simulink model "task3"  (R2023b)
settings: Solver=FixedStepDiscrete  StartTime=0.0  StopTime=10.0  FixedStep=5e-5  RelTol=1e-3
PreLoadFcn:
  | Simulink.defineIntEnumType('windowCommand', {'Off','Speed1','Speed2','Speed3'},[0,1,2,3])
libraries: simulink x1, fuzblock x1, slctrl_autotuning x1, slpidlib x1
settings Model: Creator=kz1nz0  LastModifiedBy=Ja

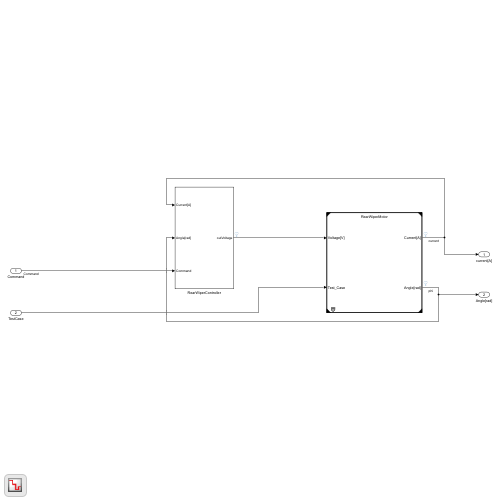
[thumbnail: Simulink's stored preview of the top-level diagram]
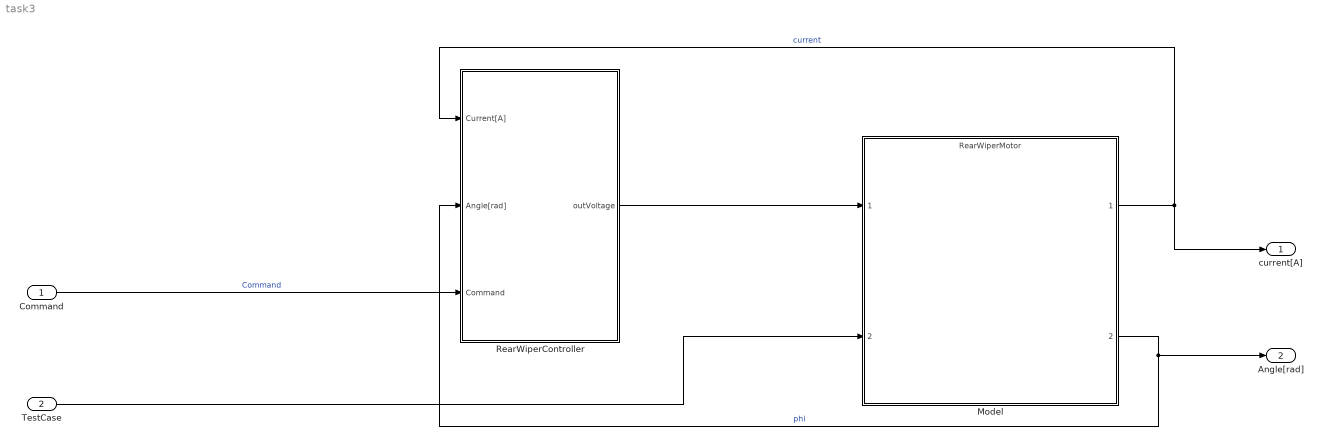
== system task3 ==
  Command : Inport  OutDataTypeStr=Enum: windowCommand
  TestCase : Inport  Port=2  OutDataTypeStr=int8
  Model : ModelReference  ModelNameDialog=RearWiperMotor.slxp  ModelReferenceVersion=19.15  CopyOfModelProtected=on
  RearWiperController : Subsystem
  current[A] : Outport
  Angle[rad] : Outport  Port=2
  wires:
  Command/1 -> RearWiperController/3(Command)  "Command"
  TestCase/1 -> Model/2
  Model/1 -> current[A]/1, RearWiperController/1(Current[A])  "current"
  Model/2 -> RearWiperController/2(Angle[rad]), Angle[rad]/1  "phi"
  RearWiperController/1(outVoltage) -> Model/1

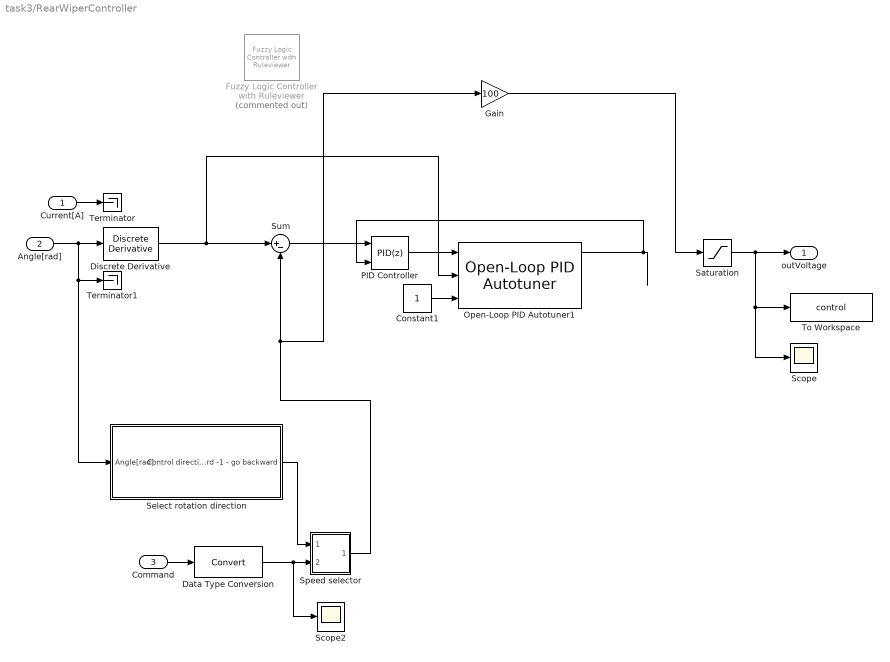
== system task3/RearWiperController ==
  Current[A] : Inport
  Angle[rad] : Inport  Port=2
  Command : Inport  Port=3  OutDataTypeStr=Enum: windowCommand
  Constant1 : Constant
  Data Type Conversion : DataTypeConversion  SaturateOnIntegerOverflow=off  RndMeth=Floor
  Discrete Derivative : simulink/Quick Insert/Discrete/Discrete Derivative  gainval=1.0  ICPrevScaledInput=0.0  OutMin=[]  OutMax=[]  OutDataType=fixdt(1, 16)  OutScaling=2^-10  DoSatur=off
  Fuzzy Logic Controller with Ruleviewer : fuzblock/Fuzzy Logic  Controller  with Ruleviewer  Commented=on  fismatrix=fis  Ts=2
  Gain : Gain  Gain=100
  Open-Loop PID Autotuner1 : slctrl_autotuning/Open-Loop PID Autotuner  PIDType=PID  PIDForm=Parallel  TimeDomain=discrete-time  DiscreteTs=5e-5  IntegratorFormula=Forward Euler  FilterFormula=Forward Euler  ContinuousTs=0.02  Bandwidth=1  UseExternalWC=off  TargetPM=60  UseExternalPM=off  UseExternalAchievedPM=off  AmpSine=1  UseExternalAmpSine=off  EstimateDCGain=on  AmpStep=1  UseExternalAmpStep=off  UseExternalFRD=off  UseExternalU0=off  UseExternalDCGain=off  NotDeployTuningModule=off  UsePLCCoder=off  BlockDataType=double  UseConnectedPID=on  blockpath=[]  tunedP=0  tunedI=0  tunedD=0  tunedN=100  tunedPM=0  EstimationWindowSize=3
      settings: LibrarySourceBlock=slctrlblks/Autotuning/Open-Loop PID Autotuner
  PID Controller : slpidlib/PID Controller  Controller=PID  Form=Parallel  TimeDomain=Discrete-time  UseExternalTs=off  SampleTime=-1  IntegratorMethod=Forward Euler  FilterMethod=Forward Euler  ControllerParametersSource=internal  P=100  I=1  UseKiTs=off  D=1  N=100  UseFilter=on  TunerSelectOption=Transfer Function Based (PID Tuner App)  InitialConditionSource=internal  InitialConditionForIntegrator=0  InitialConditionForFilter=0  DifferentiatorICPrevScaledInput=0  ExternalReset=none  TrackingMode=on  Kt=1  LimitOutput=off  SatLimitsSource=internal  UpperSaturationLimit=inf  LowerSaturationLimit=-inf  LinearizeAsGain=on  AntiWindupMode=none  Kb=1  LimitIntegrator=off  UpperIntegratorSaturationLimit=inf  LowerIntegratorSaturationLimit=-inf  POutMin=[]  POutMax=[]  IOutMin=[]  IOutMax=[]  DOutMin=[]  DOutMax=[]  NOutMin=[]  NOutMax=[]  SumOutMin=[]  SumOutMax=[]  SaturationOutMin=[]  SaturationOutMax=[]  PParamMin=[]  PParamMax=[]  IParamMin=[]  IParamMax=[]  DParamMin=[]  DParamMax=[]  NParamMin=[]  NParamMax=[]  KbParamMin=[]  KbParamMax=[]  KtParamMin=[]  KtParamMax=[]  KbOutMin=[]  KbOutMax=[]  KtOutMin=[]  KtOutMax=[]  IntegratorOutMin=[]  IntegratorOutMax=[]  FilterOutMin=[]  FilterOutMax=[]  SumI1OutMin=[]  SumI1OutMax=[]  SumI2OutMin=[]  SumI2OutMax=[]  SumI3OutMin=[]  SumI3OutMax=[]  SumI4OutMin=[]  SumI4OutMax=[]  SumDOutMin=[]  SumDOutMax=[]  DifferentiatorOutMin=[]  DifferentiatorOutMax=[]  FilterDiffOutCoefMin=[]  FilterDiffOutCoefMax=[]  ReciprocalOutMin=[]  ReciprocalOutMax=[]  SumDenOutMin=[]  SumDenOutMax=[]  SumNumOutMin=[]  SumNumOutMax=[]  DivideOutMin=[]  DivideOutMax=[]  UdiffTsProdOutMin=[]  UdiffTsProdOutMax=[]  NTsProdOutMin=[]  NTsProdOutMax=[]  UintegralTsProdOutMin=[]  UintegralTsProdOutMax=[]  UngainTsProdOutMin=[]  UngainTsProdOutMax=[]  ClampingZeroOutDataTypeStr=Inherit: Inherit via back propagation  ClampingZeroOutMin=[]  ClampingZeroOutMax=[]  FilterDenConstantOutDataTypeStr=Inherit: Inherit via back propagation  FilterDenConstantOutMin=[]  FilterDenConstantOutMax=[]  PCopyOutDataTypeStr=Inherit: Inherit via back propagation  PCopyOutMin=[]  PCopyOutMax=[]  NCopyOutDataTypeStr=Inherit: Inherit via back propagation  NCopyOutMin=[]  NCopyOutMax=[]  IntegratorContinuousStateAttributes=''  IntegratorStateMustResolveToSignalObject=off  IntegratorRTWStateStorageClass=Auto  FilterContinuousStateAttributes=''  FilterStateMustResolveToSignalObject=off  FilterRTWStateStorageClass=Auto  ParallelPVariant=InternalParameters  IdealPVariant=Disabled  IVariant=InternalParameters  DVariant=InternalParameters  IntegratorVariant=Discrete  SatVariant=Disabled  AWVariant=Passthrough  PCopyVariant=Disabled  TRVariant=Enabled  FdbkBlocksVariant=Forward  IdealPFdbkVariant=Disabled  SatFdbkVariant=Disabled  DerivativeFilterVariant=ForwardEulerFilter  NVariant=InternalParameters  NCopyVariant=Disabled  FilterICVariant=InternalICsFilter  IntegratorICVariant=InternalICs  ExternalResetVariant=Disabled  TRSumVariant=TrackingMode  SumFdbkVariant=Disabled  SumVariant=Sum_PID  TsampFilterVariant=InternalTs  TsampNgainVariant=Passthrough  TsampIntegralVariant=Disabled_SignalSpec  ExternalSaturationOutDataTypeStr=Inherit: Same as second input
  Saturation : Saturate  UpperLimit=12  LowerLimit=-12
  Scope : Scope
  Scope2 : Scope
  Select rotation direction : Subsystem
  Speed selector : Subsystem
  Sum : Sum  Inputs=|+-
  Terminator : Terminator
  Terminator1 : Terminator
  To Workspace : ToWorkspace  VariableName=control  SaveFormat=Timeseries  SampleTime=-1
  outVoltage : Outport
  wires:
  Command/1 -> Data Type Conversion/1
  Current[A]/1 -> Terminator/1
  Angle[rad]/1 -> Discrete Derivative/1, Select rotation direction/1(Angle[rad]), Terminator1/1
  Saturation/1 -> Scope/1, To Workspace/1, outVoltage/1
  Discrete Derivative/1 -> Open-Loop PID Autotuner1/2, Sum/1
  Sum/1 -> PID Controller/1
  Select rotation direction/1(Control direction 1 - go forward -1 - go backward) -> Speed selector/1(In1)
  Data Type Conversion/1 -> Scope2/1, Speed selector/2(In2)
  Open-Loop PID Autotuner1/1 -> PID Controller/2
  Speed selector/1(Out1) -> Gain/1, Sum/2
  Constant1/1 -> Open-Loop PID Autotuner1/3
  PID Controller/1 -> Open-Loop PID Autotuner1/1
  Gain/1 -> Saturation/1

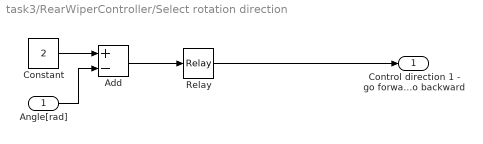
== system task3/RearWiperController/Select rotation direction ==
  Angle[rad] : Inport
  Add : Sum  Inputs=+-
  Constant : Constant  Value=2
  Relay : Relay  OnSwitchValue=1  OffSwitchValue=0  OffOutputValue=-1
  Control direction 1 - go forward -1 - go backward : Outport
  wires:
  Angle[rad]/1 -> Add/2
  Relay/1 -> Control direction 1 - go forward -1 - go backward/1
  Constant/1 -> Add/1
  Add/1 -> Relay/1

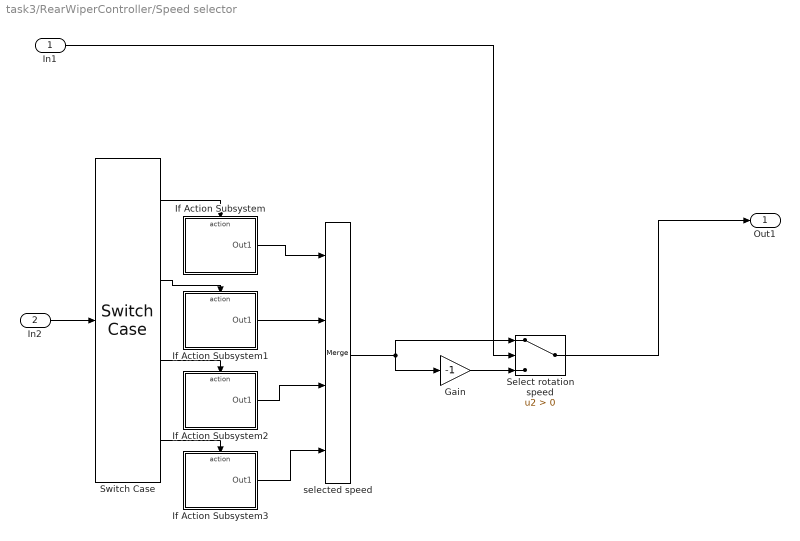
== system task3/RearWiperController/Speed selector ==
  In1 : Inport
  In2 : Inport  Port=2
  Gain : Gain  Gain=-1
  If Action Subsystem : Subsystem  TreatAsAtomicUnit=on
  If Action Subsystem1 : Subsystem  TreatAsAtomicUnit=on
  If Action Subsystem2 : Subsystem  TreatAsAtomicUnit=on
  If Action Subsystem3 : Subsystem  TreatAsAtomicUnit=on
  Select rotation speed : Switch  Criteria=u2 > Threshold  SaturateOnIntegerOverflow=off  InputSameDT=off
  Switch Case : SwitchCase  CaseConditions={1, 2, 3}
  selected speed : Merge  Inputs=4
  Out1 : Outport
  wires:
  Switch Case/3 -> If Action Subsystem2/Action
  If Action Subsystem/1(Out1) -> selected speed/1
  Switch Case/2 -> If Action Subsystem1/Action
  If Action Subsystem2/1(Out1) -> selected speed/3
  Switch Case/4 -> If Action Subsystem3/Action
  If Action Subsystem1/1(Out1) -> selected speed/2
  Switch Case/1 -> If Action Subsystem/Action
  If Action Subsystem3/1(Out1) -> selected speed/4
  Gain/1 -> Select rotation speed/3
  selected speed/1 -> Select rotation speed/1, Gain/1
  In2/1 -> Switch Case/1
  Select rotation speed/1 -> Out1/1
  In1/1 -> Select rotation speed/2

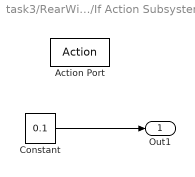
== system task3/RearWiperController/Speed selector/If Action Subsystem ==
  Action Port : ActionPort  ActionPortLabel=case [ 1 ]:
  Constant : Constant  Value=0.1
  Out1 : Outport
  wires:
  Constant/1 -> Out1/1

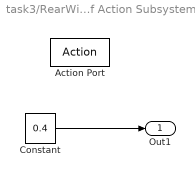
== system task3/RearWiperController/Speed selector/If Action Subsystem1 ==
  Action Port : ActionPort  ActionPortLabel=case [ 2 ]:
  Constant : Constant  Value=0.4
  Out1 : Outport
  wires:
  Constant/1 -> Out1/1

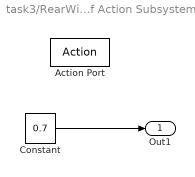
== system task3/RearWiperController/Speed selector/If Action Subsystem2 ==
  Action Port : ActionPort  ActionPortLabel=case [ 3 ]:
  Constant : Constant  Value=0.7
  Out1 : Outport
  wires:
  Constant/1 -> Out1/1

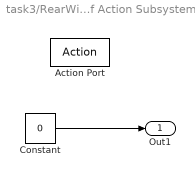
== system task3/RearWiperController/Speed selector/If Action Subsystem3 ==
  Action Port : ActionPort  ActionPortLabel=default:
  Constant : Constant  Value=0
  Out1 : Outport
  wires:
  Constant/1 -> Out1/1
